simulink model "Lab1_parameter_estimation_student"  (R2025b)
settings: Solver=FixedStepAuto  StartTime=0.0  StopTime=100  FixedStep=0.001  RelTol=1e-3
values from neighbouring files (symbols this model uses):
  motor_B = B(index)    [Lab1_motor_params_student.m]
  motor_Eff = Eff(index)    [Lab1_motor_params_student.m]
  motor_J = Jm(index)    [Lab1_motor_params_student.m]
  motor_Ke = Ke(index)    [Lab1_motor_params_student.m]
  motor_L = 0.003    [Lab1_motor_params_student.m]
  motor_R = 3.58    [Lab1_motor_params_student.m]
libraries: simulink x4, eeStairGenerator x2
settings Model: Creator=tanawatp  LastModifiedBy=ItsMoa
settings DataIOCC: OutputOption=AdditionalOutputTimes  OutputTimes=SDO_OutputTimes  ReturnWorkspaceOutputsName=SDOSimTest_Log
settings RTWCC: GPUComputeCapability=3.5

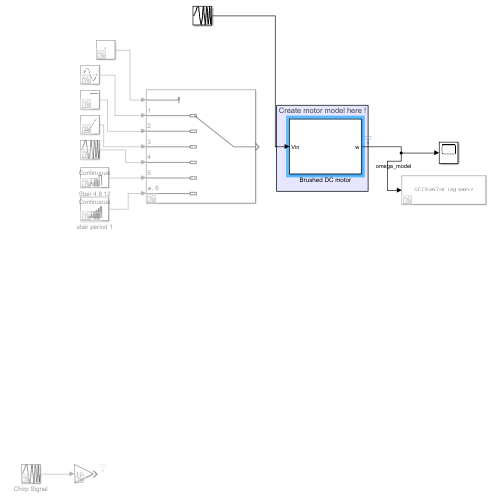
[thumbnail: Simulink's stored preview of the top-level diagram]
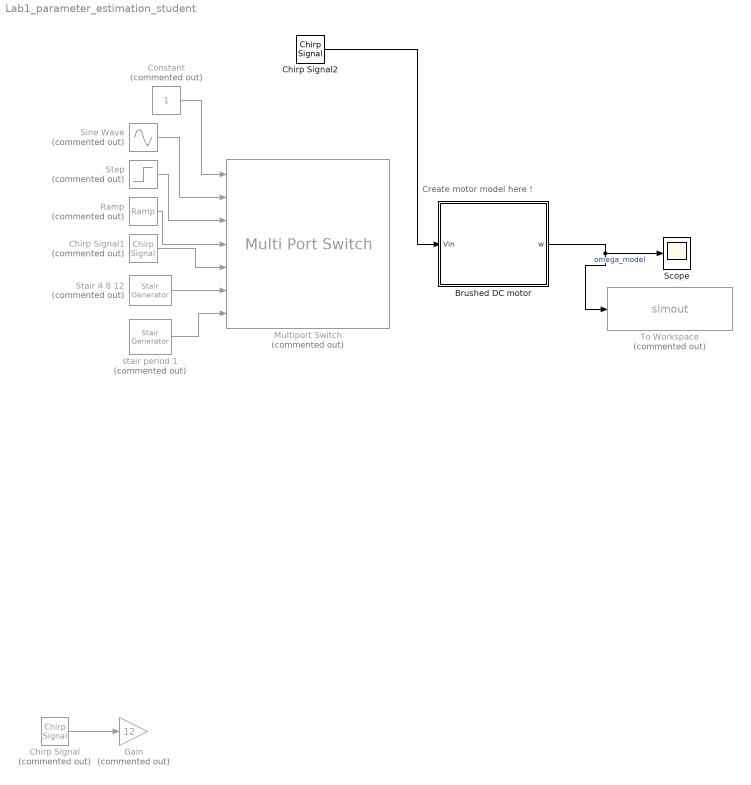
== system Lab1_parameter_estimation_student ==
  note: Create motor model here !
  Brushed DC motor : Subsystem
  Chirp Signal : simulink/Sources/Chirp Signal  Commented=on  f1=0.1  T=40  f2=5
  Chirp Signal1 : simulink/Sources/Chirp Signal  Commented=on  f1=0.1  T=30  f2=pi/2
  Chirp Signal2 : simulink/Sources/Chirp Signal  f1=0  T=50  f2=0.5
  Constant : Constant  Commented=on
  Gain : Gain  Commented=on  Gain=12
  Multiport Switch : MultiPortSwitch  Commented=on  Inputs=6  SaturateOnIntegerOverflow=off  InputSameDT=off
  Ramp : simulink/Sources/Ramp  Commented=on  slope=3  start=1  InitialOutput=0
  Scope : Scope
      settings: ActiveDisplayYMinimum=-255.35179432487251  ActiveDisplayYMaximum=259.11200055082764
  Sine Wave : Sin  Commented=on  Amplitude=12  Frequency=pi  SampleTime=0
  Stair 4 8 12 : eeStairGenerator/Stair Generator  Commented=on  LabelModeActiveChoice=Continuous  TimeInput=[0 1 2 3 4 5 6]  AmplitudeInput=[0 4 0 8 0 12 0]  SampleTime=0  RepeatPattern=off  OutDataTypeStr=double
      settings: LibrarySourceBlock=ee_sl_lib/General Control/Stair Generator
  Step : Step  Commented=on  Time=9  SampleTime=0
  To Workspace : ToWorkspace  Commented=on  VariableName=simout  SaveFormat=Timeseries  SampleTime=-1
  stair period 1 : eeStairGenerator/Stair Generator  Commented=on  LabelModeActiveChoice=Continuous  TimeInput=[0 1 2 3 4 5 6 7 8 9 10 11 12]  AmplitudeInput=[0 2 0 4 0 6 0 8 0 10 0 12 0]  SampleTime=0  RepeatPattern=off  OutDataTypeStr=double
      settings: LibrarySourceBlock=ee_sl_lib/General Control/Stair Generator
  wires:
  Brushed DC motor/1(w) -> To Workspace/1, Scope/1  "omega_model"
  Chirp Signal/1 -> Gain/1
  Constant/1 -> Multiport Switch/1
  Sine Wave/1 -> Multiport Switch/2
  Step/1 -> Multiport Switch/3
  Ramp/1 -> Multiport Switch/4
  Chirp Signal1/1 -> Multiport Switch/5
  Stair 4 8 12/1 -> Multiport Switch/6
  stair period 1/1 -> Multiport Switch/7
  Chirp Signal2/1 -> Brushed DC motor/1(Vin)

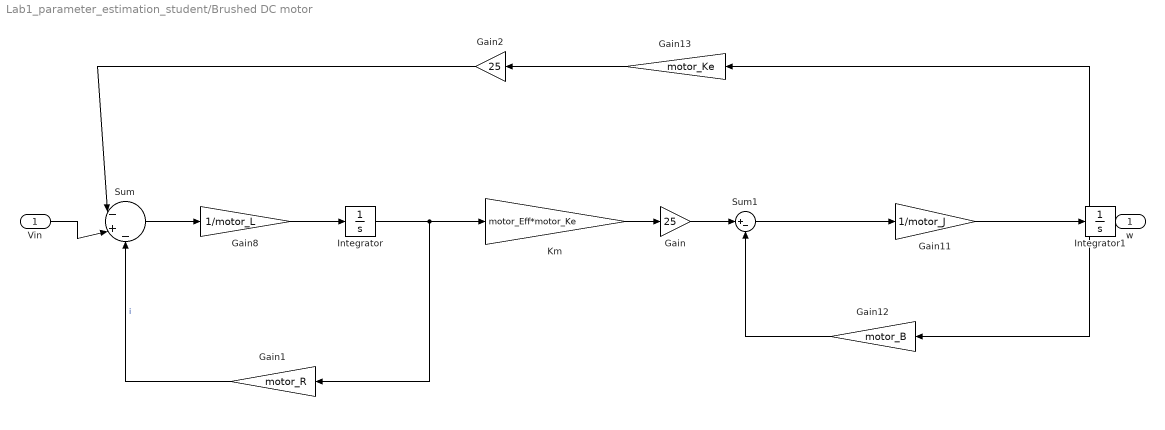
== system Lab1_parameter_estimation_student/Brushed DC motor ==
  Vin : Inport
  Gain : Gain  Gain=25
  Gain1 : Gain  Gain=motor_R
  Gain11 : Gain  Gain=1/motor_J
  Gain12 : Gain  Gain=motor_B
  Gain13 : Gain  Gain=motor_Ke
  Gain2 : Gain  Gain=25
  Gain8 : Gain  Gain=1/motor_L
  Integrator : Integrator
  Integrator1 : Integrator
  Km : Gain  Gain=motor_Eff*motor_Ke
  Sum : Sum  Inputs=|-+-
  Sum1 : Sum  Inputs=|+-
  w : Outport
  wires:
  Vin/1 -> Sum/2
  Sum/1 -> Gain8/1
  Gain8/1 -> Integrator/1
  Integrator/1 -> Gain1/1, Km/1
  Km/1 -> Gain/1
  Sum1/1 -> Gain11/1
  Gain11/1 -> Integrator1/1
  Integrator1/1 -> Gain12/1, Gain13/1, w/1
  Gain13/1 -> Gain2/1
  Gain12/1 -> Sum1/2
  Gain1/1 -> Sum/3  "i"
  Gain2/1 -> Sum/1
  Gain/1 -> Sum1/1
